simulink model "speedgoat_test_SN5659_R2021b_IO503"  (R2021b)
settings: Solver=FixedStepDiscrete  StartTime=0.0  StopTime=20  RelTol=1e-3
PreLoadFcn:
  | Ts_IO107 = 0.001;
  | Ts_IO107 = 0.001;
  | Ts_IO133 = 0.001
  | 
  | Ts_IO204 = 0.001;
  | 
  | 
  | Ts_IO503 = 0.01;
  | 
  | ts_IO612 = 1e-3;
  | Ts_IO682 = 0.005;
  | Ts_IO941 = 0.01;
InitFcn:
  | Ts_IO107 = 0.001;
  | Ts_IO107 = 0.001;
  | Ts_IO133 = 0.001
  | 
  | Ts_IO204 = 0.001;
  | 
  | 
  | Ts_IO503 = 0.01;
  | 
  | ts_IO612 = 1e-3;
  | Ts_IO682 = 0.005;
  | Ts_IO941 = 0.01;
StopFcn:
  | if isfile(['sdi_view_',bdroot,'.mldatx'])
  |  Simulink.sdi.clearPreferences();
  |  Simulink.sdi.view();
  |  pause(3);
  |  Simulink.sdi.loadView(['sdi_view_',bdroot,]);
  | end
undefined symbols (not defined in the file): standard
libraries: slrealtimeseriallib x16, speedgoatlib_serial x9, simulink x1
settings Model: Creator=yannick.orgas  LastModifiedBy=ACH
settings SolverCC: ConcurrentTasks=on  AlgebraicLoopSolver=TrustRegion  PositivePriorityOrder=on
settings DataIOCC: LimitDataPoints=on  SaveFormat=StructureWithTime
settings OptimizationCC: BlockReduction=off  OptimizeBlockIOStorage=off
settings DebuggingCC: TasksWithSamePriorityMsg=none  UnconnectedInputMsg=none  UnconnectedOutputMsg=none  UnconnectedLineMsg=none  SFMachineParentedDataDiag=warning
settings HardwareCC: ProdBitPerLong=64  ProdLongLongMode=on  ProdHWDeviceType=Intel->x86-64 (Linux 64)
settings RTWCC: Description=Simulink Real-Time  SystemTargetFile=slrealtime.tlc  TemplateMakefile=slrealtime_default_tmf  Toolchain=Simulink Real-Time Toolchain  BuildConfiguration=Faster Runs  CodeExecutionProfiling=on  TargetLang=C++
settings SimulinkRealTimeTargetCC: UseGCCFastMath=on

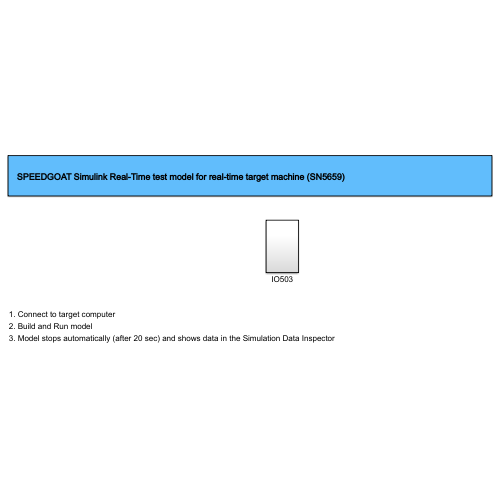
[thumbnail: Simulink's stored preview of the top-level diagram]
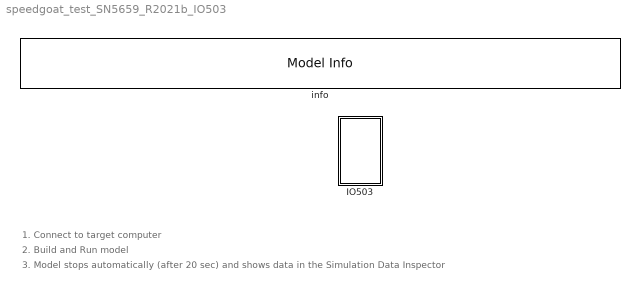
== system speedgoat_test_SN5659_R2021b_IO503 ==
  note: 1. Connect to target computer
  note: 2. Build and Run model
  note: 3. Model stops automatically (after 20 sec) and shows data in the Simulation Data Inspector
  IO503 : Subsystem
  info : simulink/Model-Wide Utilities/Model Info  Frame=on  DisplayStringWithTags=SPEEDGOAT Simulink Real-Time test model for real-time target machine (SN5659)  HorizontalTextAlignment=Left  LeftAlignmentValue=0.02

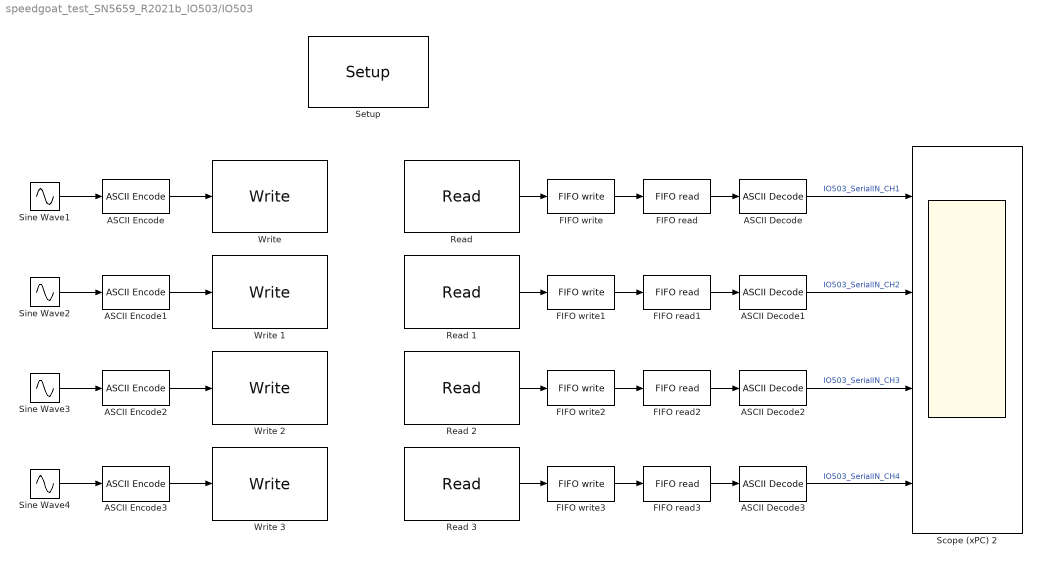
== system speedgoat_test_SN5659_R2021b_IO503/IO503 ==
  ASCII Decode{,1..3} (4 alike) : slrealtimeseriallib/ASCII Decode  format=%f\r  nvars=1  vartypes={'double'}
      settings: SourceProductBaseCode=XP
  ASCII Encode{,1..3} (4 alike) : slrealtimeseriallib/ASCII Encode  format=%f\r  nvars=1  maxlength=64  vartypes={ 'double' }
      settings: SourceProductBaseCode=XP
  FIFO read{,1..3} (4 alike) : slrealtimeseriallib/FIFO read  maxsize=64  minsize=1  usedelimiter=on  delimiter=13  outputtype=8 bit uint null terminated  enable=off  enableout=off  sampletime=Ts_IO503
      settings: SourceProductBaseCode=XP
  FIFO write : slrealtimeseriallib/FIFO write  size=64  inputtype=count+32 bit uint  present=off  sampletime=-1  id=Rx Ch1 overflow
      settings: SourceProductBaseCode=XP
  FIFO write1 : slrealtimeseriallib/FIFO write  size=64  inputtype=count+32 bit uint  present=off  sampletime=-1  id=Rx Ch2 overflow
      settings: SourceProductBaseCode=XP
  FIFO write2 : slrealtimeseriallib/FIFO write  size=64  inputtype=count+32 bit uint  present=off  sampletime=-1  id=Rx Ch3 overflow
      settings: SourceProductBaseCode=XP
  FIFO write3 : slrealtimeseriallib/FIFO write  size=64  inputtype=count+32 bit uint  present=off  sampletime=-1  id=Rx Ch4 overflow
      settings: SourceProductBaseCode=XP
  "Read " : speedgoatlib_serial/Speedgoat Shared blocks/Read   parModuleType=IO503  parModuleId=1  parChannel=1  parSampleTime=Ts_IO503  parFlush=on  parEnLegacy=on  parDataType=count+32 bit uint  parSlot=-1  parRxSwFifoSize=64
  Read 1 : speedgoatlib_serial/Speedgoat Shared blocks/Read   parModuleType=IO503  parModuleId=1  parChannel=2  parSampleTime=Ts_IO503  parFlush=on  parEnLegacy=on  parDataType=count+32 bit uint  parSlot=-1  parRxSwFifoSize=64
  Read 2 : speedgoatlib_serial/Speedgoat Shared blocks/Read   parModuleType=IO503  parModuleId=1  parChannel=3  parSampleTime=Ts_IO503  parFlush=on  parEnLegacy=on  parDataType=count+32 bit uint  parSlot=-1  parRxSwFifoSize=64
  Read 3 : speedgoatlib_serial/Speedgoat Shared blocks/Read   parModuleType=IO503  parModuleId=1  parChannel=4  parSampleTime=Ts_IO503  parFlush=on  parEnLegacy=on  parDataType=count+32 bit uint  parSlot=-1  parRxSwFifoSize=64
  "Scope (xPC) 2 " : Scope  NumInputPorts=4
  "Setup " : speedgoatlib_serial/Speedgoat Shared blocks/Setup   parModuleType=IO503  parModuleId=1  parSlot=-1  parTransceiver1=RS232  parTransceiver2=RS232  parTransceiver3=RS422  parTransceiver4=RS422  parTransceiver5=RS232  parTransceiver6=RS232  parTransceiver7=RS232  parTransceiver8=RS232  parTxTerm1=off  parRxTerm1=off  parMessageMonitoring1=off  parAutoTurnaround1=off  parTurnaroundDelay1=0  parStandardBaud1=on  parBaudrate1=921600  parBaudDivisor1=1  parSamplingRate1=16x (standard)  parPrescale1=off  parCalcBaud1=2764800  parParity1=None  parDataBits1=8  parStopBits1=1  parTxTrigLvl1=1  parRxTrigLvl1=8  parHandshake1=none  parRtsHysteresis1=0  parXon1=17  parXoff1=19  parTxSwFifoSize1=64  parRxSwFifoSize1=64  parTxTerm2=off  parRxTerm2=off  parMessageMonitoring2=off  parAutoTurnaround2=off  parTurnaroundDelay2=0  parStandardBaud2=on  parBaudrate2=921600  parBaudDivisor2=1  parSamplingRate2=16x (standard)  parPrescale2=off  parCalcBaud2=2764800  parParity2=None  parDataBits2=8  parStopBits2=1  parTxTrigLvl2=1  parRxTrigLvl2=8  parHandshake2=none  parRtsHysteresis2=0  parXon2=17  parXoff2=19  parTxSwFifoSize2=64  parRxSwFifoSize2=64  parTxTerm3=off  parRxTerm3=on  parMessageMonitoring3=off  parAutoTurnaround3=off  parTurnaroundDelay3=0  parStandardBaud3=on  parBaudrate3=2764800  parBaudDivisor3=1  parSamplingRate3=16x (standard)  parPrescale3=off  parCalcBaud3=2764800  parParity3=None  parDataBits3=8  parStopBits3=1  parTxTrigLvl3=1  parRxTrigLvl3=8  parHandshake3=none  parRtsHysteresis3=0  parXon3=17  parXoff3=19  parTxSwFifoSize3=64  parRxSwFifoSize3=64  parTxTerm4=off  parRxTerm4=on  parMessageMonitoring4=off  parAutoTurnaround4=off  parTurnaroundDelay4=0  parStandardBaud4=on  parBaudrate4=2764800  parBaudDivisor4=1  parSamplingRate4=16x (standard)  parPrescale4=off  parCalcBaud4=2764800  parParity4=None  parDataBits4=8  parStopBits4=1  parTxTrigLvl4=1  parRxTrigLvl4=8  parHandshake4=none  parRtsHysteresis4=0  parXon4=17  parXoff4=19  parTxSwFifoSize4=64  parRxSwFifoSize4=64  parTxTerm5=off  parRxTerm5=off  parMessageMonitoring5=off  parAutoTurnaround5=off  parTurnaroundDelay5=0  parStandardBaud5=on  parBaudrate5=115200  parBaudDivisor5=1  parSamplingRate5=16x (standard)  parPrescale5=off  parCalcBaud5=2764800  parParity5=None  parDataBits5=8  parStopBits5=1  parTxTrigLvl5=1  parRxTrigLvl5=1  parHandshake5=none  parRtsHysteresis5=0  parXon5=17  parXoff5=19  parTxSwFifoSize5=1024  parRxSwFifoSize5=1024  parTxTerm6=off  parRxTerm6=off  parMessageMonitoring6=off  parAutoTurnaround6=off  parTurnaroundDelay6=0  parStandardBaud6=on  parBaudrate6=115200  parBaudDivisor6=1  parSamplingRate6=16x (standard)  parPrescale6=off  parCalcBaud6=2764800  parParity6=None  parDataBits6=8  parStopBits6=1  parTxTrigLvl6=1  parRxTrigLvl6=1  parHandshake6=none  parRtsHysteresis6=0  parXon6=17  parXoff6=19  parTxSwFifoSize6=1024  parRxSwFifoSize6=1024  parTxTerm7=off  parRxTerm7=off  parMessageMonitoring7=off  parAutoTurnaround7=off  parTurnaroundDelay7=0  parStandardBaud7=on  parBaudrate7=115200  parBaudDivisor7=1  parSamplingRate7=16x (standard)  parPrescale7=off  parCalcBaud7=2764800  parParity7=None  parDataBits7=8  parStopBits7=1  parTxTrigLvl7=1  parRxTrigLvl7=1  parHandshake7=none  parRtsHysteresis7=0  parXon7=17  parXoff7=19  parTxSwFifoSize7=1024  parRxSwFifoSize7=1024  parTxTerm8=off  parRxTerm8=off  parMessageMonitoring8=off  parAutoTurnaround8=off  parTurnaroundDelay8=0  parStandardBaud8=on  parBaudrate8=115200  parBaudDivisor8=1  parSamplingRate8=16x (standard)  parPrescale8=off  parCalcBaud8=2764800  parParity8=None  parDataBits8=8  parStopBits8=1  parTxTrigLvl8=1  parRxTrigLvl8=1  parHandshake8=none  parRtsHysteresis8=0  parXon8=17  parXoff8=19  parTxSwFifoSize8=1024  parRxSwFifoSize8=1024
      settings: SourceProductName=Simulink Real-Time: Speedgoat I/O Driver Library
  Sine Wave1 : Sin  Amplitude=10  Bias=127  Frequency=1*2*pi  SampleTime=Ts_IO503
  Sine Wave2 : Sin  Amplitude=20  Bias=127  Frequency=1*2*pi  SampleTime=Ts_IO503
  Sine Wave3 : Sin  Amplitude=30  Bias=127  Frequency=1*2*pi  SampleTime=Ts_IO503
  Sine Wave4 : Sin  Amplitude=40  Bias=127  Frequency=1*2*pi  SampleTime=Ts_IO503
  "Write " : speedgoatlib_serial/Speedgoat Shared blocks/Write   parModuleType=IO503  parModuleId=1  parChannel=1  parSampleTime=-1  parEnLegacy=on  parDataType=8 bit uint null terminated  parSlot=-1  parTxSwFifoSize=64
  Write 1 : speedgoatlib_serial/Speedgoat Shared blocks/Write   parModuleType=IO503  parModuleId=1  parChannel=2  parSampleTime=-1  parEnLegacy=on  parDataType=8 bit uint null terminated  parSlot=-1  parTxSwFifoSize=64
  Write 2 : speedgoatlib_serial/Speedgoat Shared blocks/Write   parModuleType=IO503  parModuleId=1  parChannel=3  parSampleTime=-1  parEnLegacy=on  parDataType=8 bit uint null terminated  parSlot=-1  parTxSwFifoSize=64
  Write 3 : speedgoatlib_serial/Speedgoat Shared blocks/Write   parModuleType=IO503  parModuleId=1  parChannel=4  parSampleTime=-1  parEnLegacy=on  parDataType=8 bit uint null terminated  parSlot=-1  parTxSwFifoSize=64
  wires:
  Sine Wave4/1 -> ASCII Encode3/1
  Sine Wave3/1 -> ASCII Encode2/1
  Sine Wave1/1 -> ASCII Encode/1
  Sine Wave2/1 -> ASCII Encode1/1
  ASCII Decode/1 -> "Scope (xPC) 2 "/1  "IO503_SerialIN_CH1"
  ASCII Decode1/1 -> "Scope (xPC) 2 "/2  "IO503_SerialIN_CH2"
  ASCII Decode2/1 -> "Scope (xPC) 2 "/3  "IO503_SerialIN_CH3"
  ASCII Decode3/1 -> "Scope (xPC) 2 "/4  "IO503_SerialIN_CH4"
  FIFO write/1 -> FIFO read/1
  "Read "/1 -> FIFO write/1
  FIFO write1/1 -> FIFO read1/1
  Read 1/1 -> FIFO write1/1
  FIFO write2/1 -> FIFO read2/1
  FIFO write3/1 -> FIFO read3/1
  FIFO read1/1 -> ASCII Decode1/1
  FIFO read2/1 -> ASCII Decode2/1
  FIFO read3/1 -> ASCII Decode3/1
  Read 2/1 -> FIFO write2/1
  Read 3/1 -> FIFO write3/1
  ASCII Encode/1 -> "Write "/1
  FIFO read/1 -> ASCII Decode/1
  ASCII Encode1/1 -> Write 1/1
  ASCII Encode2/1 -> Write 2/1
  ASCII Encode3/1 -> Write 3/1
